simulink model "f-dev"  (R2021b)
settings: Solver=VariableStepAuto  StartTime=0.0  StopTime=10.0  RelTol=1e-3
settings Model: Creator=schae  LastModifiedBy=schae

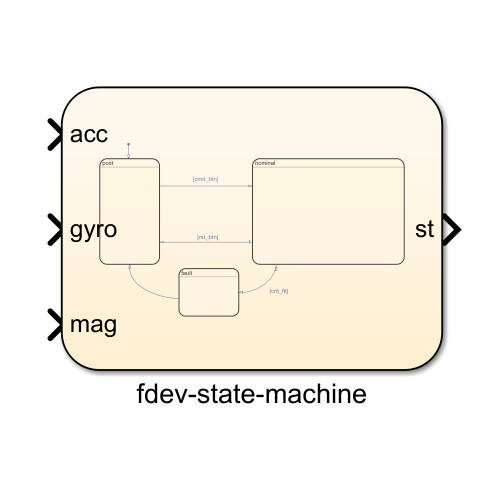
[thumbnail: Simulink's stored preview of the top-level diagram]
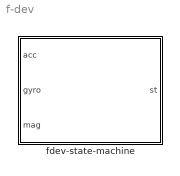
== system f-dev ==
  fdev-state-machine : Stateflow chart  TreatAsAtomicUnit=on

== stateflow chart f-dev/fdev-state-machine ==
  state post/
    state startup/
      st = 0;
    (default) -> startup
  state nominal/
    state idle/
      st = 10;
    state in_motion/
      st = 11;
    state landed/
      st = 13;
    state flying/
      st = 12;
    (default) -> idle
    idle -> in_motion : [v > v_thr]
    landed -> idle
    in_motion -> flying : [v > v_thr && w >= w_thr]
    flying -> landed : [v < v_thr && w <= w_thr]
  state fault/
    state faulted/
      st = -1;
    (default) -> faulted
  (default) -> post
  post -> nominal : [cmd_btn]
  nominal -> post [order 1] : [rst_btn]
  fault -> post
  nominal -> fault [order 2] : [crit_flt]
  data: acc input; gyro input; mag input; st output
